simulink model "modulation_delay"  (Simulink 4.00)
settings: Solver=ode45  StartTime=0.0  StopTime=100  RelTol=1e-3
undefined symbols (not defined in the file): slcm
libraries: commdigbbndpm2 x2, commchan2 x1, commsink2 x1, commsource2 x1
settings Model: LastModifiedBy=agaltman  BlockReductionOpt=off

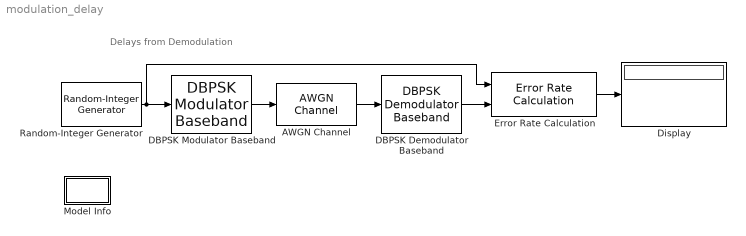
== system modulation_delay ==
  note: Delays from Demodulation
  AWGN Channel : commchan2/AWGN Channel  seed=1237  noiseMode="Signal to noise ratio  (Es/No)"  EsNodB=4  SNRdB=10  Ps=1  Tsym=1  variance=1
  DBPSK Demodulator Baseband : commdigbbndpm2/DBPSK Demodulator Baseband  Ph=0  numSamp=8
  DBPSK Modulator Baseband : commdigbbndpm2/DBPSK Modulator Baseband  Ph=0  numSamp=8
  Display : Display
      settings: Format=short
  Error Rate Calculation : commsink2/Error Rate Calculation  N=1  st_delay=1  cp_mode=Entire frame  subframe=[]  PMode=Port  WsName=ErrorVec  RsMode2=off
  Model Info : Subsystem  LoadFcn=slcm LoadBlock;  InitFcn=slcm('UpdateAllCMBlocksInThisModelInit')  mask(CMBlock){InitialSaveTempField=, InitialBlockCM=none, BlockCM=none, Frame=on, SaveTempField=, DisplayStringWithTags=Info, MaskDisplayString=Info, HorizontalTextAlignment=Center, LeftAlignmentValue=0.5, SourceBlockDiagram=modulation_delay, TagMaxNumber=20, CMTag1=, CMTag2=, CMTag3=, CMTag4=, CMTag5=, CMTag6=, CMTag7=, CMTag8=, CMTag9=, CMTag10=, CMTag11=, CMTag12=, CMTag13=, CMTag14=, CMTag15=, CMTag16=, CMTag17=, CMTag18=, CMTag19=, CMTag20=}
      mask help: This block allows revision control information to be displayed within the model.
      settings: CopyFcn=slcm CopyBlock;  DeleteFcn=slcm Cancel;  PostSaveFcn=slcm('UpdateAllCMBlocksInThisModel')  NameChangeFcn=slcm Rename;  OpenFcn=commdemohelp;  RTWFcnNameOpts=Auto  RTWFileNameOpts=Auto
      mask Display: text(str2num(LeftAlignmentValue), 0.5, MaskDisplayString, 'HorizontalAlignment', HorizontalTextAlignment)
  Random-Integer Generator : commsource2/Random-Integer Generator  mul=2  seed=10711  Ts=1  frameBased=off  sampPerFrame=1  orient=off
  wires:
  Random-Integer Generator/1 -> Error Rate Calculation/1, DBPSK Modulator Baseband/1
  DBPSK Modulator Baseband/1 -> AWGN Channel/1
  DBPSK Demodulator Baseband/1 -> Error Rate Calculation/2
  Error Rate Calculation/1 -> Display/1
  AWGN Channel/1 -> DBPSK Demodulator Baseband/1

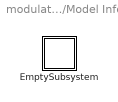
== system modulation_delay/Model Info ==
  EmptySubsystem : Subsystem
      settings: RTWFcnNameOpts=Auto  RTWFileNameOpts=Auto

== system modulation_delay/Model Info/EmptySubsystem ==
